simulink model "HVAC_Ctrl_V1_1"  (R2018a)
settings: configuration reference "Configuration" (kept outside this file)
PreLoadFcn:
  | HVAC_Ctrl_V1_BusInfo
libraries: simulink x2
settings Model: Creator=IAEC nishito  LastModifiedBy=E00026
settings ConfigSetRef: SourceLocation=Base Workspace

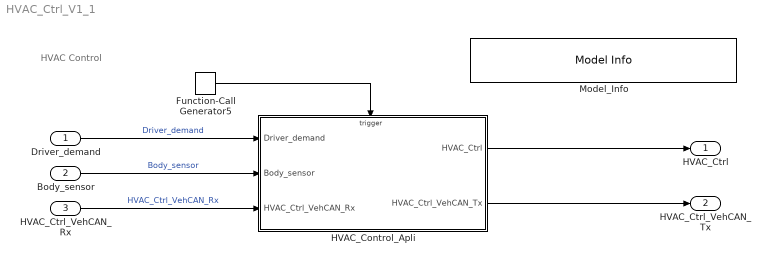
== system HVAC_Ctrl_V1_1 ==
  note: HVAC Control
  Driver_demand : Inport  OutDataTypeStr=Bus: Driver_demand_Bus
      settings: AttributesFormatString=<%<OutDataTypeStr>>
  Body_sensor : Inport  Port=2  OutDataTypeStr=Bus: Body_sensor_Bus
      settings: AttributesFormatString=<%<OutDataTypeStr>>
  HVAC_Ctrl_VehCAN_Rx : Inport  Port=3  OutDataTypeStr=Bus: HVAC_Ctrl_VehCAN_Rx_Bus
      settings: AttributesFormatString=<%<OutDataTypeStr>>
  Function-Call Generator5 : simulink/Ports & Subsystems/Function-Call Generator  sample_time=0.05  numberOfIterations=1
      settings: AttributesFormatString=<sample_time=%<sample_time>>
  HVAC_Control_Apli : Subsystem
  Model_Info : simulink/Model-Wide Utilities/Model Info  Frame=on  DisplayStringWithTags=|  HorizontalTextAlignment=Left  LeftAlignmentValue=0.02
      | Version  %<ModelVersion>
      | LastModifided by %<LastModifiedBy>  Date %<LastModificationDate>
      | Description  %<Description>
  HVAC_Ctrl : Outport  OutDataTypeStr=Bus: HVAC_Ctrl_Bus
      settings: AttributesFormatString=<%<OutDataTypeStr>>
  HVAC_Ctrl_VehCAN_Tx : Outport  Port=2  OutDataTypeStr=Bus: HVAC_Ctrl_VehCAN_Tx_Bus
      settings: AttributesFormatString=<%<OutDataTypeStr>>
  wires:
  HVAC_Control_Apli/2(HVAC_Ctrl_VehCAN_Tx) -> HVAC_Ctrl_VehCAN_Tx/1
  HVAC_Ctrl_VehCAN_Rx/1 -> HVAC_Control_Apli/3(HVAC_Ctrl_VehCAN_Rx)  "HVAC_Ctrl_VehCAN_Rx"
  Driver_demand/1 -> HVAC_Control_Apli/1(Driver_demand)  "Driver_demand"
  HVAC_Control_Apli/1(HVAC_Ctrl) -> HVAC_Ctrl/1
  Function-Call Generator5/1 -> HVAC_Control_Apli/Trigger
  Body_sensor/1 -> HVAC_Control_Apli/2(Body_sensor)  "Body_sensor"

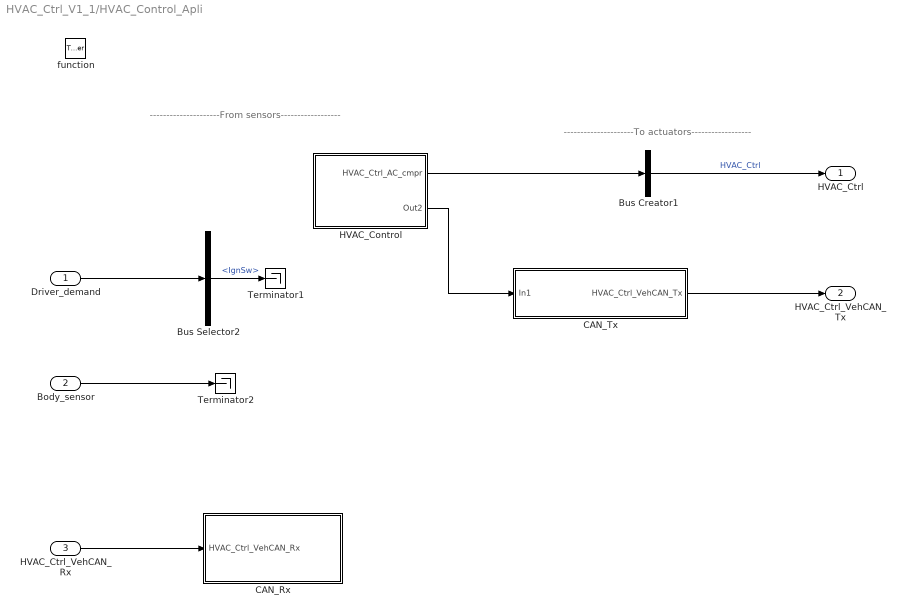
== system HVAC_Ctrl_V1_1/HVAC_Control_Apli ==
  note: ---------------------From sensors------------------
  note: ---------------------To actuators------------------
  Driver_demand : Inport
  Body_sensor : Inport  Port=2
  HVAC_Ctrl_VehCAN_Rx : Inport  Port=3
  function : TriggerPort  TriggerType=function-call  VariantControl=Variant
  Bus Creator1 : BusCreator  Inputs=1  OutDataTypeStr=Bus: HVAC_Ctrl_Bus
      settings: AttributesFormatString=<%<OutDataTypeStr>>
  Bus Selector2 : BusSelector  OutputSignals=IgnSw
  CAN_Rx : Subsystem
  CAN_Tx : Subsystem
  HVAC_Control : Subsystem
  Terminator1 : Terminator
  Terminator2 : Terminator
  HVAC_Ctrl : Outport
  HVAC_Ctrl_VehCAN_Tx : Outport  Port=2
  wires:
  Driver_demand/1 -> Bus Selector2/1
  Bus Creator1/1 -> HVAC_Ctrl/1  "HVAC_Ctrl"
  Body_sensor/1 -> Terminator2/1
  Bus Selector2/1 -> Terminator1/1  "<IgnSw>"
  CAN_Tx/1(HVAC_Ctrl_VehCAN_Tx) -> HVAC_Ctrl_VehCAN_Tx/1
  HVAC_Ctrl_VehCAN_Rx/1 -> CAN_Rx/1(HVAC_Ctrl_VehCAN_Rx)
  HVAC_Control/1(HVAC_Ctrl_AC_cmpr) -> Bus Creator1/1
  HVAC_Control/2(Out2) -> CAN_Tx/1(In1)

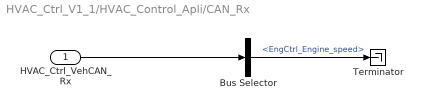
== system HVAC_Ctrl_V1_1/HVAC_Control_Apli/CAN_Rx ==
  HVAC_Ctrl_VehCAN_Rx : Inport
  Bus Selector : BusSelector  OutputSignals=EngCtrl_Engine_speed
  Terminator : Terminator
  wires:
  Bus Selector/1 -> Terminator/1  "<EngCtrl_Engine_speed>"
  HVAC_Ctrl_VehCAN_Rx/1 -> Bus Selector/1

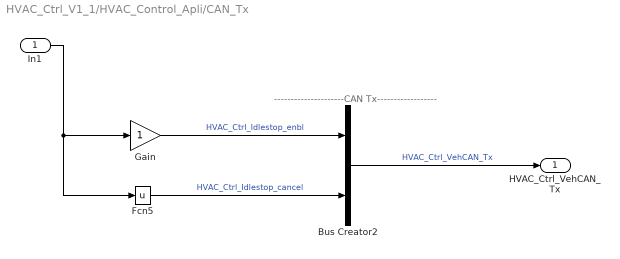
== system HVAC_Ctrl_V1_1/HVAC_Control_Apli/CAN_Tx ==
  note: ---------------------CAN Tx------------------
  In1 : Inport
  Bus Creator2 : BusCreator  Inputs=2  OutDataTypeStr=Bus: HVAC_Ctrl_VehCAN_Tx_Bus
      settings: AttributesFormatString=<%<OutDataTypeStr>>
  Fcn5 : Fcn  Expr=u
  Gain : Gain
  HVAC_Ctrl_VehCAN_Tx : Outport
  wires:
  In1/1 -> Gain/1, Fcn5/1
  Gain/1 -> Bus Creator2/1  "HVAC_Ctrl_Idlestop_enbl"
  Fcn5/1 -> Bus Creator2/2  "HVAC_Ctrl_Idlestop_cancel"
  Bus Creator2/1 -> HVAC_Ctrl_VehCAN_Tx/1  "HVAC_Ctrl_VehCAN_Tx"

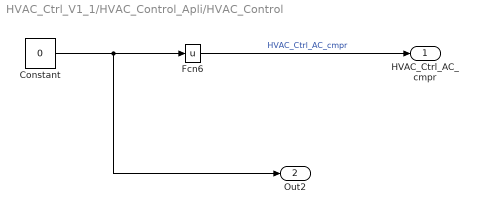
== system HVAC_Ctrl_V1_1/HVAC_Control_Apli/HVAC_Control ==
  Constant : Constant  Value=0
  Fcn6 : Fcn  Expr=u
  HVAC_Ctrl_AC_cmpr : Outport
  Out2 : Outport  Port=2
  wires:
  Constant/1 -> Out2/1, Fcn6/1
  Fcn6/1 -> HVAC_Ctrl_AC_cmpr/1  "HVAC_Ctrl_AC_cmpr"
